simulink model "Plant"  (R2020b)
settings: Solver=VariableStepAuto  StartTime=0.0  StopTime=10.0  RelTol=1e-3
values from neighbouring files (symbols this model uses):
  plant_den = [1 1/50.5355]    [Headway_Controller_Design.m]
  plant_num = 9.22123*1e-4    (= 0.000922123)    [Headway_Controller_Design.m]
settings Model: Creator=ChOm1  LastModifiedBy=ChOm1

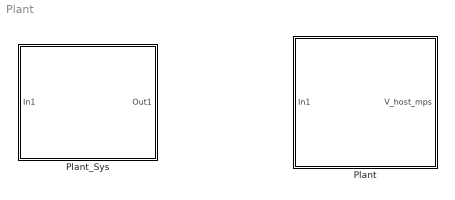
== system Plant ==
  Plant : Subsystem
  Plant_Sys : Subsystem

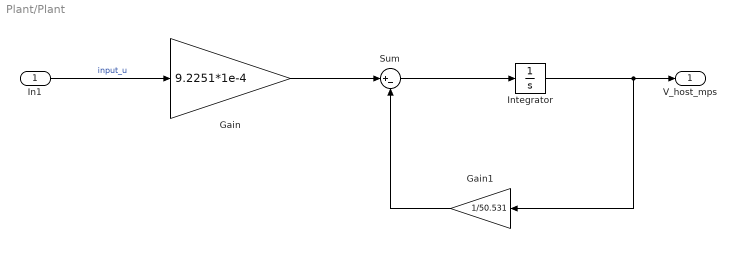
== system Plant/Plant ==
  In1 : Inport
  Gain : Gain  Gain=9.2251*1e-4
  Gain1 : Gain  Gain=1/50.531
  Integrator : Integrator
  Sum : Sum  Inputs=|+-
  V_host_mps : Outport
  wires:
  In1/1 -> Gain/1  "input_u"
  Gain/1 -> Sum/1
  Sum/1 -> Integrator/1
  Integrator/1 -> Gain1/1, V_host_mps/1
  Gain1/1 -> Sum/2

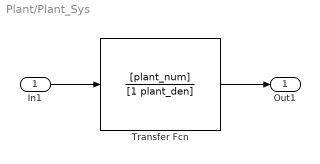
== system Plant/Plant_Sys ==
  In1 : Inport
  Transfer Fcn : TransferFcn  Numerator=[plant_num]  Denominator=[1 plant_den]
  Out1 : Outport
  wires:
  In1/1 -> Transfer Fcn/1
  Transfer Fcn/1 -> Out1/1
